simulink model "Sim_Rate_Limiters_iqctest"  (Simulink 7.3)
settings: Solver=ode45  StartTime=0.0  StopTime=20.0  RelTol=1e-3
settings Model: Creator=MD710  LastModifiedBy=MD710
settings DebuggingCC: SaveWithParameterizedLinksMsg=none  SolverPrmCheckMsg=none  MultiTaskDSMMsg=warning  MultiTaskCondExecSysMsg=none  FcnCallInpInsideContextMsg=Enable All  StrictBusMsg=None
settings HardwareCC: TargetHWDeviceType=32-bit Generic
settings RTWCC: IncludeERTFirstTime=on
settings GRTTargetCC: TargetFcnLib=ansi_tfl_tmw.mat

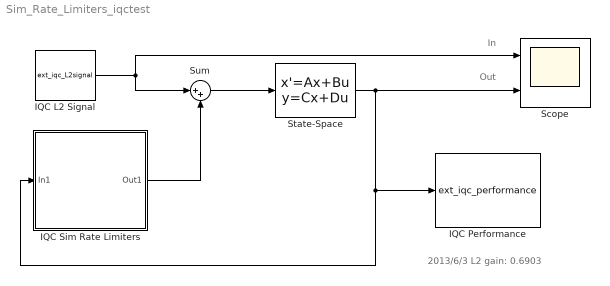
== system Sim_Rate_Limiters_iqctest ==
  note: 2013/6/3 L2 gain: 0.6903
  note: In
  note: Out
  IQC L2 Signal : M-S-Function  FunctionName=ext_iqc_L2signal  Parameters=sig_size,sam_time,sig_type,tru_time,sig_amp,sig_fre,user_cus  mask(IQC L2 signal(ver:0.1)){sig_size=1, sam_time=0, sig_type=Step, tru_time=10, sig_amp=1, sig_fre=1, user_cus='2*exp(3*t)'}
      mask prompts: sig_size "Signal Dimension:(Default: 1)"; sam_time "Sample Time:(Default: 0)"; sig_type "Signal Type:"; tru_time "Truncation Time:"; sig_amp "Maximum Amplitude:"; sig_fre "Frequency:"; user_cus "Custom:"
      mask help:
      | Important:
      | In IQC procedure step (as commond iqc_gain_tbx, the task is get
      | L2 gain value), regardless of the user to choose which option (ex sine...),
      | here regarded as generalized L2 signal.
      mask StyleString: edit,edit,popup(Step|Square wave|Sine wave|Custom|Random|External),edit,edit,edit,edit
      mask CallbackString: ||iqc_block_cho(gcb,'L2signal_type')||||
      mask TabNameString: Main,Main,Simulation,Simulation,Simulation,Simulation,Simulation
      mask Display: plot(0:0.1:10,[sin(0:0.1:6.2) zeros(1,38)])
  IQC Performance : M-S-Function  FunctionName=ext_iqc_performance  Parameters=imp_met,save_lin_com,isiqcbode,fre_ran,uselmitool,lmi_par  mask(IQC Performance(ver:0.1)){imp_met=Calculation and Simulation, save_lin_com=off, isiqcbode=off, fre_ran='', uselmitool=lmilab, lmi_par=''}
      mask prompts: imp_met "Implementation Methods"; save_lin_com "Save the Linear File and Command File"; isiqcbode "Display IQC Bode Figure"; fre_ran "Frequency Range:(Default: empty)"; uselmitool "LMI Tool:"; lmi_par "Parameter:(if empty use define)"
      mask help:
      | Important:
      | In IQC toolbox calculate step (as commond iqc_gain_tbx, the task is get
      | L2 gain value), regardless of the user to connect any signal input(Even if
      | not a signal), here regarded as generalized L2 signal.
      |
      | Example 1: setlmioptions('',[0 200 0 0 777])
      | the block parameter is
      | LMI Tool: lmilab
      | Parameter:
      |        [0 200 0 0 777]
      |
      | Example 2: setlmioptions('yalmip','solver','sdpt3','verbose',1)
      | the block parameter is
      | LMI Tool: yalmip
      | Parameter:
      |        {'solver',sdpt3','verbose',1}
      mask Help:
      | <a href="matlab:doc abst_init_iqc;">abst_init_iqc</a>
      | <a href="matlab:doc setlmioptions;">setlmioptions</a>
      | <a href="matlab:doc iqc_gain_tbx;">iqc_gain_tbx</a>
      mask StyleString: popup(Calculation and Simulation|Only Calculation|Only Simulation),checkbox,checkbox,edit,popup(lmilab|yalmip),edit
      mask CallbackString: iqc_block_cho(gcb,'performance_imp')||iqc_block_cho(gcb,'performance_bodefre')|||
      mask TabNameString: Main,Main,Main,Main,LMI,LMI
      mask Display: fprintf('In -> Out \n performance \n L2 gain:\n%4.4f',0.69027);
  IQC Sim Rate Limiters : Subsystem  mask(IQC Sim Rate Limiters(ver:0.1)){upp_lim=1, low_lim=-1, d_sat=1, firstpole=1, iqc1=on, iqc1_pole=[1], iqc1_out='', iqc2=off, lis_rel=''}
      mask prompts: upp_lim "Upper Limit of Saturation:"; low_lim "Lower Limit of Saturation:"; d_sat "Slope of Saturation:(Default: 1)"; firstpole "(s+Pole1) ~ the Pole1:(Default: 1)"; iqc1 "iqc_ratelimiter(Input,[Pole1 Pole],Slope)  (only for scalar input)"; iqc1_pole "Pole:(Default: [1])"; iqc1_out "Output Variable:(Default: empty)"; iqc2 "Custom IQC"; lis_rel "List of IQC Relationships:"
      mask init:
      | if length(firstpole)>1
      |     error('the Pole1 only scalar')
      | end
      | if length(d_sat)>1
      |     error('d(Sat(0))/dt only scalar')
      | end
      mask Help: <a href="matlab:doc iqc_ratelimiter;">iqc_ratelimiter</a>
      mask CallbackString: ||||iqc_block_cho(gcb,'sim_ratelim_iqc1')|||iqc_block_cho(gcb,'sim_ratelim_iqc2')|
      mask TabNameString: Simulink Parameters,Simulink Parameters,Simulink Parameters,Simulink Parameters,Procedure Parameters,Procedure Parameters,Procedure Parameters,Procedure Parameters,Procedure Parameters
      mask Display: plot(0,0,100,100,[18,45,45,18,18],[60,60,26,26,60],[62,82,82,62,62],[60,60,26,26,60],[62,0],[44,44],[79,65],[44,44],[71,71],[46,57],[68,69,72,74,73,71,69,68,69,72,74],[31,29,29,31,34,35,36,38,40,40,39],[31,31],[26,60],[45,38,24],[55,55,33],[24,18],[33,33],[99,82],[44,44],[10,12,8,10,10,90,90],[44,51,51,44,80,80,44],[7,2],[55,55])
  Scope : Scope  NumInputPorts=2
      settings: YMin=-5~-5  YMax=5~5
  State-Space : StateSpace  A=[-5,1;2,-3]  B=[0;1]  C=[0 1]  D=[0]
  Sum : Sum  Inputs=|++
  wires:
  Sum/1 -> State-Space/1
  IQC Sim Rate Limiters/1(Out1) -> Sum/2
  IQC L2 Signal/1 -> Sum/1, Scope/1
  State-Space/1 -> IQC Sim Rate Limiters/1(In1), IQC Performance/1, Scope/2

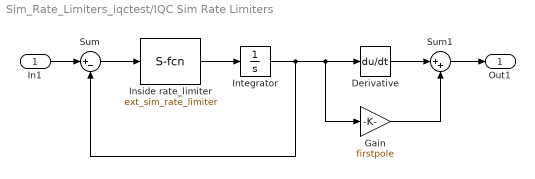
== system Sim_Rate_Limiters_iqctest/IQC Sim Rate Limiters ==
  In1 : Inport
  Derivative : Derivative
  Gain : Gain  Gain=firstpole
  Inside rate_limiter : M-S-Function  FunctionName=ext_sim_rate_limiter  Parameters=upp_lim,low_lim,d_sat,firstpole,iqc1,iqc1_pole,iqc1_out,iqc2,lis_rel
  Integrator : Integrator
  Sum : Sum  Inputs=|+-
  Sum1 : Sum  Inputs=|++
  Out1 : Outport
  wires:
  In1/1 -> Sum/1
  Sum1/1 -> Out1/1
  Sum/1 -> Inside rate_limiter/1
  Integrator/1 -> Sum/2, Derivative/1, Gain/1
  Inside rate_limiter/1 -> Integrator/1
  Derivative/1 -> Sum1/1
  Gain/1 -> Sum1/2
